simulink model "LMI"  (R2025b)
settings: Solver=VariableStepAuto  StartTime=0.0  StopTime=10.0  RelTol=1e-3
undefined symbols (not defined in the file): A, B, C, Comp, D, h0, h_ref, K2
settings Model: Creator=inggi  LastModifiedBy=inggi

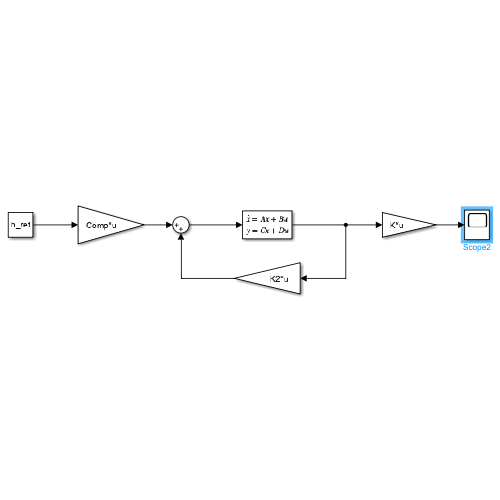
[thumbnail: Simulink's stored preview of the top-level diagram]
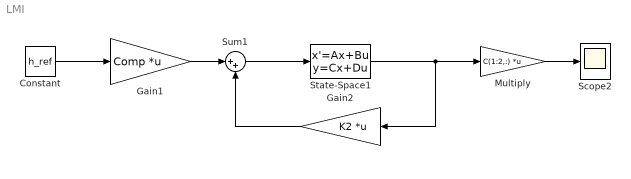
== system LMI ==
  Constant : Constant  Value=h_ref
  Gain1 : Gain  Gain=Comp  Multiplication=Matrix(K*u)
  Gain2 : Gain  Gain=K2  Multiplication=Matrix(K*u)
  Multiply : Gain  Gain=C(1:2,:)  Multiplication=Matrix(K*u)
  Scope2 : Scope
      settings: ActiveDisplayYMinimum=0.15764283179027108  ActiveDisplayYMaximum=0.55465719635945332  DataLoggingVariableName=ScopeData2
  State-Space1 : StateSpace  A=A  B=B  C=C  D=D  InitialCondition=h0
  Sum1 : Sum  Inputs=|++
  wires:
  Multiply/1 -> Scope2/1
  Sum1/1 -> State-Space1/1
  Gain1/1 -> Sum1/1
  State-Space1/1 -> Multiply/1, Gain2/1
  Gain2/1 -> Sum1/2
  Constant/1 -> Gain1/1
